simulink model "Single phase Semi Converter Motor Control"  (R2024b)
settings: Solver=VariableStepAuto  StartTime=0.0  StopTime=2  MaxStep=10e-6  RelTol=1e-3
undefined symbols (not defined in the file): alpha
libraries: spsCurrentMeasurementLib x2, spsDiodeLib x2, spsThyristorLib x2, spsVoltageMeasurementLib x2, spsACVoltageSourceLib x1, spsDCMachineLib x1, spsDCVoltageSourceLib x1, sps_lib x1
settings Model: Creator=Desktop  LastModifiedBy=Rajat Dhanure

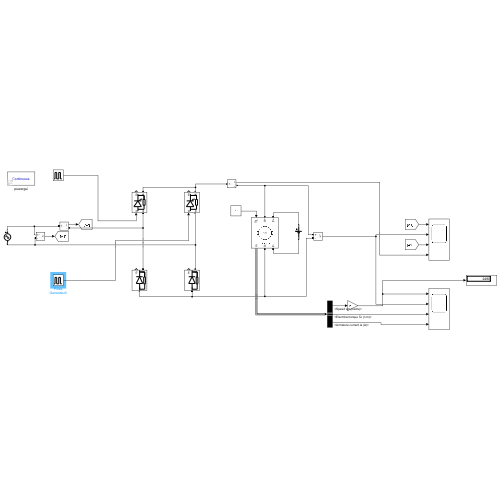
[thumbnail: Simulink's stored preview of the top-level diagram]
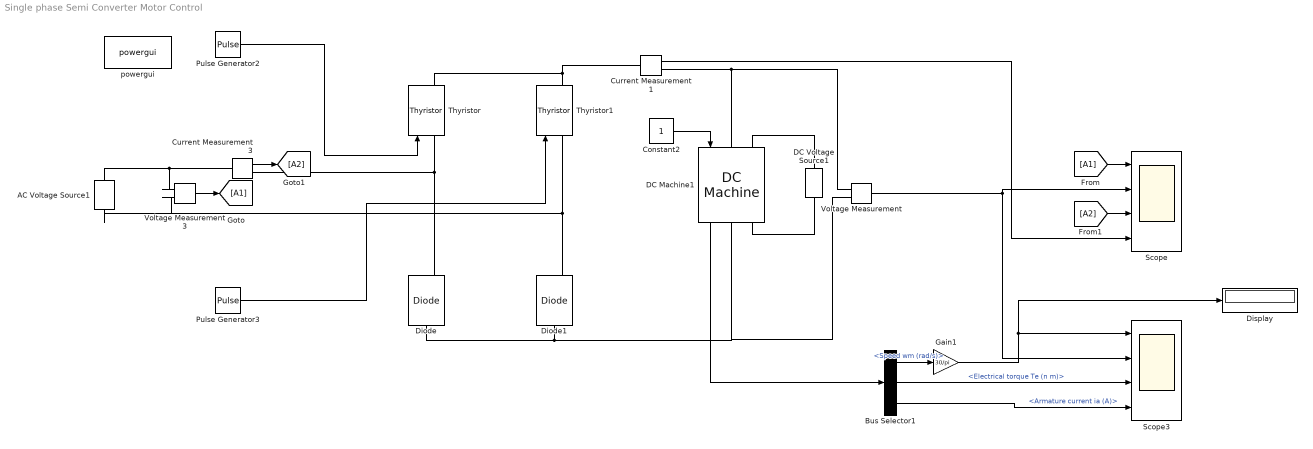
== system Single phase Semi Converter Motor Control ==
  AC Voltage Source1 : spsACVoltageSourceLib/AC Voltage Source  Amplitude=240 * sqrt(2)  Phase=0  Frequency=50  SampleTime=0  Measurements=None  BusType=swing  Pref=10e3  Qref=0  Qmin=-inf  Qmax=+inf
  Bus Selector1 : BusSelector  OutputSignals=Speed wm (rad/s),Electrical torque Te (n m),Armature current ia (A)
  Constant2 : Constant
  Current Measurement1 : spsCurrentMeasurementLib/Current Measurement  PhasorSimulation=off  OutputType=Complex  PSBequivalent=0
  Current Measurement3 : spsCurrentMeasurementLib/Current Measurement  PhasorSimulation=off  OutputType=Complex  PSBequivalent=0
  DC Machine1 : spsDCMachineLib/DC Machine  PresetModel=01: 5HP 240V 1750RPM Field:300V  MechanicalLoad=Torque TL  FieldType=Wound  ShowDetailedParameters=on  MeasurementBus=off  RLa=[2.581 0.028]  RLf=[281.2 156]  Laf=0.9483  MachineConstant=Torque constant (N.m/A)  Ke=1.8  Kt=1.8  J=0.02215  Bm=0.002953  Tf=0.5161  w0=1  Ifinit=1.06685632871799  TsPowergui=0  TsBlock=-1
  DC Voltage Source1 : spsDCVoltageSourceLib/DC Voltage Source  Amplitude=300  Measurements=None
  Diode : spsDiodeLib/Diode  Ron=0.001  Lon=0  Vf=0.8  IC=0  UseSnubber=0  Rs=500  Cs=250e-9  Measurements=on
  Diode1 : spsDiodeLib/Diode  Ron=0.001  Lon=0  Vf=0.8  IC=0  UseSnubber=0  Rs=500  Cs=250e-9  Measurements=on
  Display : Display
  Gain1 : Gain  Gain=30/pi
  Pulse Generator2 : DiscretePulseGenerator  PulseType=Time based  Period=1/50  PulseWidth=20  PhaseDelay=(1/50) * (alpha)/360
  Pulse Generator3 : DiscretePulseGenerator  PulseType=Time based  Period=1/50  PulseWidth=20  PhaseDelay=(1/50) * (180 + alpha)/360
  Scope : Scope  NumInputPorts=4
  Scope3 : Scope  NumInputPorts=4
  Thyristor : spsThyristorLib/Thyristor  Ron=0.001  Lon=0  Vf=0.8  IC=0  Rs=500  Cs=250e-9  Measurements=on
  Thyristor1 : spsThyristorLib/Thyristor  Ron=0.001  Lon=0  Vf=0.8  IC=0  Rs=500  Cs=250e-9  Measurements=on
  Voltage Measurement : spsVoltageMeasurementLib/Voltage Measurement  PhasorSimulation=off  OutputType=Complex  PSBequivalent=0
  Voltage Measurement3 : spsVoltageMeasurementLib/Voltage Measurement  PhasorSimulation=off  OutputType=Complex  PSBequivalent=0
  powergui : sps_lib/powergui  Priority=1  SimulationMode=Continuous  SampleTime=50e-6  frequency=60  Iterations=50  frequencyindice=50  Pbase=100e6  ErrMax=1e-4  UnitsV=kV  UnitsW=MW  buscounter=0  FunctionMessages=off  echomessages=off  EnableUseOfTLC=off  CurrentSourceSwitches=off  DisableSnubberDevices=off  DisableRonSwitches=off  DisableVfSwitches=off  DisplayEquations=off  AutomaticDiscreteSolvers=off  SolverType=Tustin/Backward Euler (TBE)  Interpol=off  ExternalGateDelay=off  methode=off  Ts=100  x0status=blocks  SPID=on  SwTol=0  HookPort=off  NonlinearTolerance=1e-4  nMaxIteration=100  ContinueOnMaxIteration=off  RestoreLinks=warning  ResistiveCurrentMeasurement=off  Frange=[0:2:500]  Ylog=off  Xlog=on  ShowGrid=off  save=off  variable=ZData  structure=0  ZoomFFT=off  StartTime=0.0  cycles=1  DisplayStyle=1  fundamental=60  FreqAxis=off  MaxFrequency=1000  frequencyindicesteady=1  RmsSteady=1  display=off
  wires:
  Pulse Generator2/1 -> Thyristor/1
  Pulse Generator3/1 -> Thyristor1/1
  Voltage Measurement3/1 -> [A1]
  [A1] -> Scope/1
  Current Measurement3/1 -> [A2]
  [A2] -> Scope/3
  Constant2/1 -> DC Machine1/1
  DC Machine1/1 -> Bus Selector1/1
  Bus Selector1/1 -> Gain1/1  "<Speed wm (rad/s)>"
  Gain1/1 -> Display/1, Scope3/1
  Bus Selector1/2 -> Scope3/3  "<Electrical torque Te (n m)>"
  Bus Selector1/3 -> Scope3/4  "<Armature current ia (A)>"
  Current Measurement1/1 -> Scope/4
  Voltage Measurement/1 -> Scope3/2, Scope/2
  connections:
  AC Voltage Source1/RConn1 -- Current Measurement3/LConn1 -- Voltage Measurement3/LConn1
  Voltage Measurement3/LConn2 -- AC Voltage Source1/LConn1 -- Diode1/RConn1 -- Thyristor1/LConn1
  Current Measurement1/RConn1 -- Voltage Measurement/LConn1 -- DC Machine1/LConn1
  DC Machine1/RConn1 -- Voltage Measurement/LConn2 -- Diode1/LConn1 -- Diode/LConn1
  Current Measurement3/RConn1 -- Thyristor/LConn1 -- Diode/RConn1
  DC Voltage Source1/RConn1 -- DC Machine1/LConn2
  DC Voltage Source1/LConn1 -- DC Machine1/RConn2
  Thyristor/RConn1 -- Current Measurement1/LConn1 -- Thyristor1/RConn1
